simulink model "DynamicVibrationAbsorber"  (R2020b)
settings: Solver=VariableStepAuto  StartTime=0.0  StopTime=50  RelTol=1e-3
model workspace (MAT data in the model file):
  F = 10
  d1 = 15
  d2 = 10
  k1 = 10
  k2 = 10
  m1 = 20
  m2 = 20
settings Model: OrderedModelArguments=off  Creator=Administrator  LastModifiedBy=Administrator
settings DebuggingCC: AlgebraicLoopMsg=none

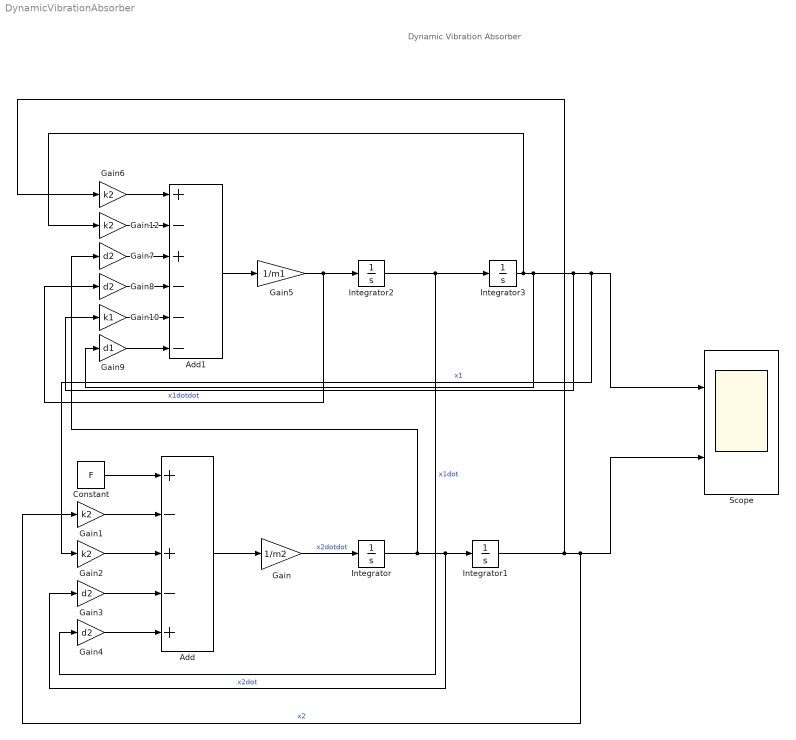
== system DynamicVibrationAbsorber ==
  note: Dynamic Vibration Absorber
  Add : Sum  Inputs=+-+-+
  Add1 : Sum  Inputs=+-+---
  Constant : Constant  Value=F
  Gain : Gain  Gain=1/m2
  Gain{1..2,6,12} (4 alike) : Gain  Gain=k2
  Gain10 : Gain  Gain=k1
  Gain{3..4,7..8} (4 alike) : Gain  Gain=d2
  Gain5 : Gain  Gain=1/m1
  Gain9 : Gain  Gain=d1
  Integrator{,1..3} (4 alike) : Integrator
  Scope : Scope  NumInputPorts=2
  wires:
  Integrator/1 -> Gain7/1, Gain3/1, Integrator1/1  "x2dot"
  Integrator1/1 -> Gain6/1, Gain1/1, Scope/2  "x2"
  Gain/1 -> Integrator/1  "x2dotdot"
  Gain5/1 -> Gain8/1, Integrator2/1  "x1dotdot"
  Integrator3/1 -> Gain12/1, Gain9/1, Gain2/1, Scope/1, Gain10/1  "x1"
  Integrator2/1 -> Gain4/1, Integrator3/1  "x1dot"
  Add/1 -> Gain/1
  Constant/1 -> Add/1
  Gain1/1 -> Add/2
  Gain2/1 -> Add/3
  Gain3/1 -> Add/4
  Gain4/1 -> Add/5
  Add1/1 -> Gain5/1
  Gain12/1 -> Add1/2
  Gain7/1 -> Add1/3
  Gain8/1 -> Add1/4
  Gain10/1 -> Add1/5
  Gain9/1 -> Add1/6
  Gain6/1 -> Add1/1
